simulink model "linearizeController"  (R2015a)
settings: Solver=ode45  StartTime=0.0  StopTime=10.0  RelTol=1e-3
undefined symbols (not defined in the file or in its folder): quad, sampleTime_qcsim
settings Model: Creator=ra  LastModifiedBy=ra

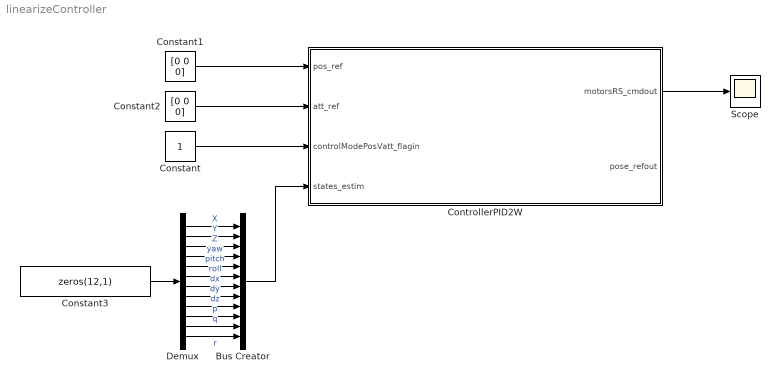
== system linearizeController ==
  Bus Creator : BusCreator  Inputs=12
  Constant : Constant
  Constant1 : Constant  Value=[0 0 0]
  Constant2 : Constant  Value=[0 0 0]
  Constant3 : Constant  Value=zeros(12,1)
  ControllerPID2W : Subsystem  TreatAsAtomicUnit=on
  Demux : Demux  Outputs=12
  Scope : Scope
      settings: SaveName=ScopeData2
  wires:
  ControllerPID2W/1(motorsRS_cmdout) -> Scope/1
  Demux/1 -> Bus Creator/1  "X"
  Demux/2 -> Bus Creator/2  "Y"
  Demux/3 -> Bus Creator/3  "Z"
  Demux/4 -> Bus Creator/4  "yaw"
  Demux/5 -> Bus Creator/5  "pitch"
  Demux/6 -> Bus Creator/6  "roll"
  Demux/7 -> Bus Creator/7  "dx"
  Demux/8 -> Bus Creator/8  "dy"
  Demux/9 -> Bus Creator/9  "dz"
  Demux/10 -> Bus Creator/10  "p"
  Demux/11 -> Bus Creator/11  "q"
  Demux/12 -> Bus Creator/12  "r"
  Constant3/1 -> Demux/1
  Bus Creator/1 -> ControllerPID2W/4(states_estim)
  Constant1/1 -> ControllerPID2W/1(pos_ref)
  Constant2/1 -> ControllerPID2W/2(att_ref)
  Constant/1 -> ControllerPID2W/3(controlModePosVatt_flagin)

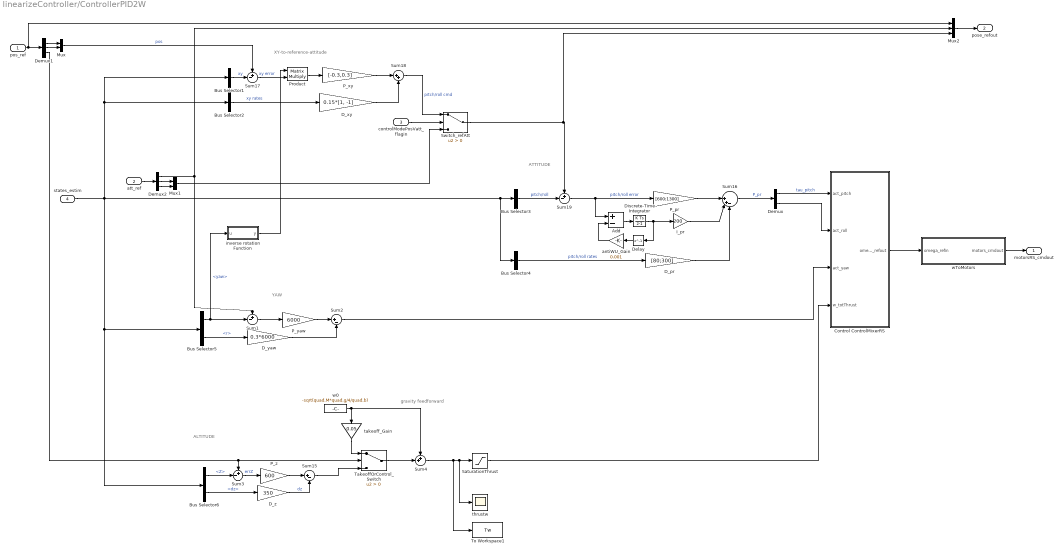
== system linearizeController/ControllerPID2W ==
  note: XY-to-reference-attitude
  note: ALTITUDE
  note: ATTITUDE
  note: YAW
  note: gravity feedforward
  pos_ref : Inport
  att_ref : Inport  Port=2
  controlModePosVatt_flagin : Inport  Port=3
  states_estim : Inport  Port=4
  Add : Sum  Inputs=+-
  Bus Selector1 : BusSelector  OutputSignals=X,Y  OutputAsBus=on
  Bus Selector2 : BusSelector  OutputSignals=dx,dy  OutputAsBus=on
  Bus Selector3 : BusSelector  OutputSignals=pitch,roll  OutputAsBus=on
  Bus Selector4 : BusSelector  OutputSignals=q,p  OutputAsBus=on
  Bus Selector5 : BusSelector  OutputSignals=yaw,r
  Bus Selector6 : BusSelector  OutputSignals=Z,dz
  Control ControlMixerRS : Subsystem
  D_pr : Gain  Gain=[80;300]
  D_xy : Gain  Gain=0.15*[1, -1]
  D_yaw : Gain  Gain=0.3*6000
  D_z : Gain  Gain=350
  Delay : Delay  DelayLength=1  InitialCondition=0
  Demux : Demux  Outputs=2
  Demux1 : Demux  Outputs=3
  Demux2 : Demux  Outputs=3
  Discrete-Time Integrator : DiscreteIntegrator  InitialConditionSetting=State (most efficient)  SampleTime=sampleTime_qcsim  LimitOutput=on  UpperSaturationLimit=2  LowerSaturationLimit=-2
  I_pr : Gain  Gain=200
  Mux : Mux  Inputs=2
  Mux1 : Mux  Inputs=2
  Mux2 : Mux  Inputs=3
  P_pr : Gain  Gain=[600;1300]
  P_xy : Gain  Gain=[-0.3,0.3]
  P_yaw : Gain  Gain=6000
  P_z : Gain  Gain=600
  Product : Product  Multiplication=Matrix(*)  RndMeth=Zero
  SaturationThrust : Saturate  UpperLimit=0.92*2618  LowerLimit=-0.92*2618
  Sum{1,3,17,19} (4 alike) : Sum  Inputs=+-|
  Sum15 : Sum  Inputs=|+-
  Sum16 : Sum  Inputs=||++-
  Sum18 : Sum  Inputs=|++
  Sum2 : Sum  Inputs=|+-
  Sum4 : Sum  Inputs=++|
  Switch_refAtt : Switch  Criteria=u2 > Threshold
  TakeoffOrControl_Switch : Switch  Criteria=u2 > Threshold
  To Workspace1 : ToWorkspace  VariableName=Tw  SampleTime=-1
  antiWU_Gain : Gain  Gain=0.001
  inverse rotation Function : MATLAB Function  TreatAsAtomicUnit=on
  takeoff_Gain : Gain  Gain=0.05
  thrustw : Scope
      settings: YMin=-0.04  YMax=0.045  SaveName=ScopeData15
  w0 : Constant  Value=-sqrt(quad.M*quad.g/4/quad.b)  SampleTime=sampleTime_qcsim
  wToMotors : Subsystem
  motorsRS_cmdout : Outport
  pose_refout : Outport  Port=2
  wires:
  w0/1 -> takeoff_Gain/1, Sum4/1
  Bus Selector2/1 -> D_xy/1  "xy rates"
  Bus Selector4/1 -> D_pr/1  "pitch/roll rates"
  Sum19/1 -> P_pr/1, Add/1  "pitch/roll error"
  Sum16/1 -> Demux/1  "P_pr"
  Bus Selector5/1 -> inverse rotation Function/1(u), Sum1/2  "<yaw>"
  Bus Selector6/1 -> Sum3/2  "<Z>"
  inverse rotation Function/1(y) -> Product/1
  Bus Selector5/2 -> D_yaw/1  "<r>"
  Sum3/1 -> P_z/1  "errZ"
  Bus Selector6/2 -> D_z/1  "<dz>"
  D_z/1 -> Sum15/2  "dz"
  D_yaw/1 -> Sum2/2
  Sum4/1 -> To Workspace1/1, thrustw/1, SaturationThrust/1
  Sum1/1 -> P_yaw/1
  Sum17/1 -> Product/2  "xy error"
  Discrete-Time Integrator/1 -> Delay/1, I_pr/1
  Demux/1 -> Control ControlMixerRS/1(act_pitch)  "tau_pitch"
  Sum2/1 -> Control ControlMixerRS/3(act_yaw)
  Demux/2 -> Control ControlMixerRS/2(act_roll)
  TakeoffOrControl_Switch/1 -> Sum4/2
  Sum15/1 -> TakeoffOrControl_Switch/3
  takeoff_Gain/1 -> TakeoffOrControl_Switch/1
  Sum18/1 -> Switch_refAtt/1  "pitch/roll cmd"
  controlModePosVatt_flagin/1 -> Switch_refAtt/2
  pos_ref/1 -> Mux2/1, Demux1/1
  Demux1/1 -> Mux/1
  Demux1/2 -> Mux/2
  Mux/1 -> Sum17/1  "pos"
  Demux2/2 -> Mux1/1
  Demux2/3 -> Mux1/2
  att_ref/1 -> Demux2/1
  Mux1/1 -> Switch_refAtt/3
  Demux2/1 -> Mux2/2, Sum1/1
  Demux1/3 -> Sum3/1, TakeoffOrControl_Switch/2
  Bus Selector3/1 -> Sum19/2  "pitch/roll"
  Product/1 -> P_xy/1
  D_xy/1 -> Sum18/2
  Bus Selector1/1 -> Sum17/2  "xy"
  P_z/1 -> Sum15/1
  SaturationThrust/1 -> Control ControlMixerRS/4(w_totThrust)
  P_yaw/1 -> Sum2/1
  I_pr/1 -> Sum16/2
  D_pr/1 -> Sum16/3
  P_pr/1 -> Sum16/1
  Control ControlMixerRS/1(omega_refout) -> wToMotors/1(omega_refin)
  wToMotors/1(motors_cmdout) -> motorsRS_cmdout/1
  Mux2/1 -> pose_refout/1
  Switch_refAtt/1 -> Mux2/3, Sum19/1
  states_estim/1 -> Bus Selector4/1, Bus Selector3/1, Bus Selector1/1, Bus Selector2/1, Bus Selector5/1, Bus Selector6/1
  P_xy/1 -> Sum18/1
  Add/1 -> Discrete-Time Integrator/1
  antiWU_Gain/1 -> Add/2
  Delay/1 -> antiWU_Gain/1

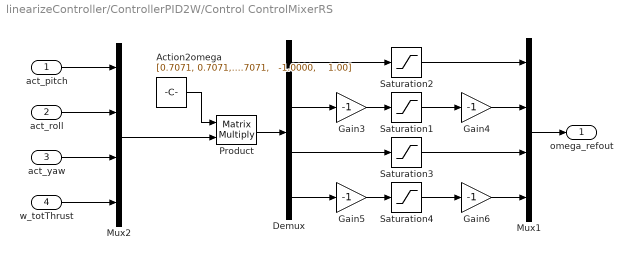
== system linearizeController/ControllerPID2W/Control ControlMixerRS ==
  act_pitch : Inport
  act_roll : Inport  Port=2
  act_yaw : Inport  Port=3
  w_totThrust : Inport  Port=4
  Action2omega : Constant  Value="[0.7071, 0.7071, -1.0000, -1.00;   -0.7071,    0.7071,   -1.0000,    1.00;   -0.7071,   -0.7071,   -1.0000,   -1.00;    0.7071,   -0.7071,   -1.0000,    1.00]"
  Demux : Demux
  Gain{3..6} (4 alike) : Gain  Gain=-1
  Mux1 : Mux
  Mux2 : Mux
  Product : Product  Multiplication=Matrix(*)  RndMeth=Zero
  Saturation{1..4} (4 alike) : Saturate  UpperLimit=2618  LowerLimit=500
  omega_refout : Outport
  wires:
  Saturation3/1 -> Mux1/3
  Saturation4/1 -> Gain6/1
  Saturation2/1 -> Mux1/1
  Mux1/1 -> omega_refout/1
  Gain3/1 -> Saturation1/1
  Saturation1/1 -> Gain4/1
  Gain4/1 -> Mux1/2
  Gain5/1 -> Saturation4/1
  Gain6/1 -> Mux1/4
  act_pitch/1 -> Mux2/1
  act_roll/1 -> Mux2/2
  act_yaw/1 -> Mux2/3
  w_totThrust/1 -> Mux2/4
  Mux2/1 -> Product/2
  Action2omega/1 -> Product/1
  Product/1 -> Demux/1
  Demux/1 -> Saturation2/1
  Demux/2 -> Gain3/1
  Demux/3 -> Saturation3/1
  Demux/4 -> Gain5/1

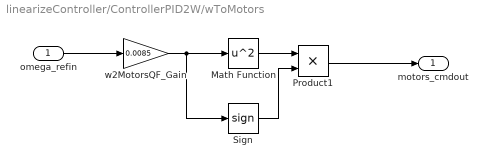
== system linearizeController/ControllerPID2W/wToMotors ==
  omega_refin : Inport
  Math Function : Math  Operator=square  SaturateOnIntegerOverflow=on
  Product1 : Product
  Sign : Signum
  w2MotorsQF_Gain : Gain  Gain=0.0085
  motors_cmdout : Outport
  wires:
  omega_refin/1 -> w2MotorsQF_Gain/1
  Math Function/1 -> Product1/1
  Product1/1 -> motors_cmdout/1
  w2MotorsQF_Gain/1 -> Sign/1, Math Function/1
  Sign/1 -> Product1/2

== matlab function linearizeController/ControllerPID2W/inverse rotation Function ==
  data: u input; y output
function y = fcn(u)
%inverse yaw-rotation
y = ([cos(u) sin(u); -sin(u) cos(u)]);
